simulink model "J8Grav_block"  (R2017b)
settings: Solver=VariableStepAuto  StartTime=0.0  StopTime=10.0  RelTol=1e-3
libraries: sharedtransform x2
settings Model: Creator=mtwal  LastModifiedBy=mtwal

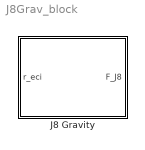
== system J8Grav_block ==
  J8 Gravity : Subsystem  mask(J8 Gravity){w_earth=0, a_earth=0, muE=0, J2_on=on, J3_on=on, J4_on=on, J5_on=on, J6_on=on, J7_on=on, J8_on=on}
      mask prompts: w_earth "Earth rotation rate"; a_earth "Earth semi-major axis"; muE "Earth gravitational parameter"; J2_on "Use J2 harmonic"; J3_on "Use J3 harmonic"; J4_on "Use J4 harmonic"; J5_on "Use J5 harmonic"; J6_on "Use J6 harmonic"; J7_on "Use J7 harmonic"; J8_on "Use J8 harmonic"
      mask help: Calculate force due to J8 gravity from inertial position

== system J8Grav_block/J8 Gravity ==
  r_eci : Inport
  Bus Creator : BusCreator  Inputs=3
  Demux : Demux  Outputs=3
  ECEF2ECI : Subsystem
  ECI2ECEF : Subsystem
  Subsystem : Subsystem
  Subsystem1 : Subsystem
  major axis : Constant  Value=a_earth
  mu : Constant  Value=muE
  F_J8 : Outport
  wires:
  r_eci/1 -> ECI2ECEF/1(v_ECI)
  ECEF2ECI/1(v_ECI) -> F_J8/1  "F_J8_ECI"
  ECI2ECEF/1(v_ECEF) -> Demux/1
  Demux/1 -> Bus Creator/1  "rx"
  Demux/2 -> Bus Creator/2  "ry"
  Demux/3 -> Bus Creator/3  "rz"
  major axis/1 -> Subsystem1/2(a_Earth)  "a_earth"
  mu/1 -> Subsystem1/3(mu_Earth)  "mu_Earth"
  Subsystem/1(J_coeff) -> Subsystem1/4(J_coeff)  "J_coeff"
  Bus Creator/1 -> Subsystem1/1(r_ECEF)  "r_ECEF"
  Subsystem1/1(F_J8Grav_ECEF) -> ECEF2ECI/1(v_ECEF)  "F_J8_ECEF"

== system J8Grav_block/J8 Gravity/ECEF2ECI ==
  v_ECEF : Inport
  Clock : Clock
  Constant : Constant  Value=0
  Gain : Gain  Gain=-w_earth
  Mux : Mux  Inputs=3
  Product : Product  Multiplication=Matrix(*)
  Rotation Angles to Direction Cosine Matrix : sharedtransform/Rotation Angles to Direction Cosine Matrix  rotationOrder=ZYX
      settings: SourceProductBaseCode=AE
  v_ECI : Outport
  wires:
  Clock/1 -> Gain/1
  Gain/1 -> Mux/1
  Product/1 -> v_ECI/1
  Rotation Angles to Direction Cosine Matrix/1 -> Product/1
  v_ECEF/1 -> Product/2
  Mux/1 -> Rotation Angles to Direction Cosine Matrix/1
  Constant/1 -> Mux/2, Mux/3

== system J8Grav_block/J8 Gravity/ECI2ECEF ==
  v_ECI : Inport
  Clock : Clock
  Constant : Constant  Value=0
  Gain : Gain  Gain=w_earth
  Mux : Mux  Inputs=3
  Product : Product  Multiplication=Matrix(*)
  Rotation Angles to Direction Cosine Matrix : sharedtransform/Rotation Angles to Direction Cosine Matrix  rotationOrder=ZYX
      settings: SourceProductBaseCode=AE
  v_ECEF : Outport
  wires:
  Clock/1 -> Gain/1
  Gain/1 -> Mux/1
  Product/1 -> v_ECEF/1
  Rotation Angles to Direction Cosine Matrix/1 -> Product/1
  v_ECI/1 -> Product/2
  Constant/1 -> Mux/2, Mux/3
  Mux/1 -> Rotation Angles to Direction Cosine Matrix/1

== system J8Grav_block/J8 Gravity/Subsystem ==
  Bus Creator : BusCreator  Inputs=7
  J2 : Subsystem
  J3 : Subsystem
  J4 : Subsystem
  J5 : Subsystem
  J6 : Subsystem
  J7 : Subsystem
  J8 : Subsystem
  J_coeff : Outport
  wires:
  J2/1(J2) -> Bus Creator/1  "J2_coeff"
  J3/1(J3) -> Bus Creator/2  "J3_coeff"
  J4/1(J4) -> Bus Creator/3  "J4_coeff"
  J5/1(J5) -> Bus Creator/4  "J5_coeff"
  J6/1(J6) -> Bus Creator/5  "J6_coeff"
  J8/1(J8) -> Bus Creator/7  "J8_coeff"
  J7/1(J7) -> Bus Creator/6  "J7_coeff"
  Bus Creator/1 -> J_coeff/1

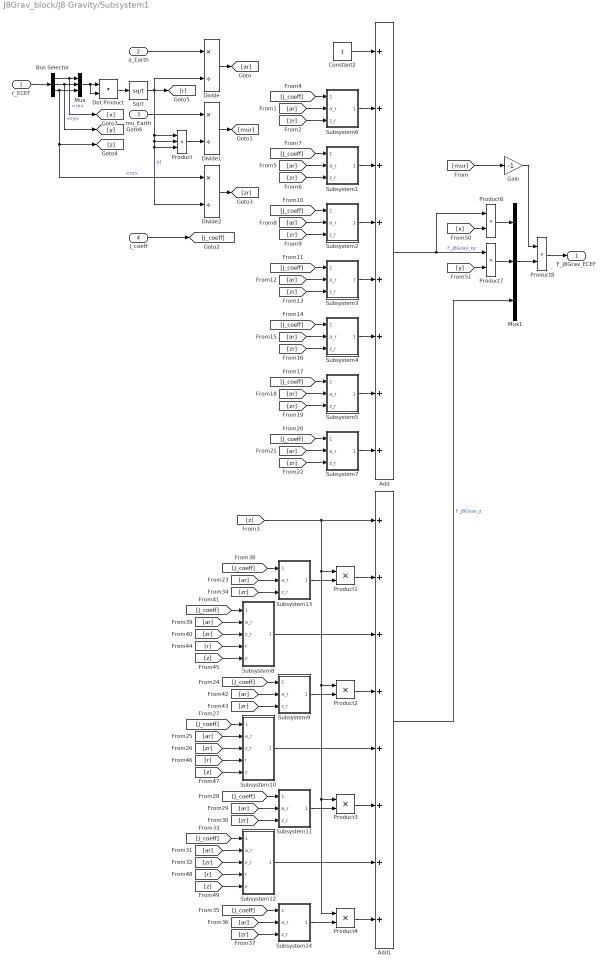
== system J8Grav_block/J8 Gravity/Subsystem1 ==
  r_ECEF : Inport
  a_Earth : Inport  Port=2
  mu_Earth : Inport  Port=3
  J_coeff : Inport  Port=4
  Add : Sum  Inputs=++++++++
  Add1 : Sum  Inputs=++++++++
  Bus Selector : BusSelector  OutputSignals=rx,ry,rz
  Constant2 : Constant
  Divide : Product  Inputs=*/
  Divide1 : Product  Inputs=*/
  Divide2 : Product  Inputs=*/
  Dot Product : DotProduct  InputSameDT=on  OutDataTypeStr=Inherit: Inherit via internal rule
  Gain : Gain  Gain=-1
  Mux : Mux  Inputs=3
  Mux1 : Mux  Inputs=3
  Product : Product  Inputs=3
  Product{1..4,6..8} (7 alike) : Product
  Sqrt : Sqrt  SaturateOnIntegerOverflow=on
  Subsystem1 : Subsystem
  Subsystem10 : Subsystem
  Subsystem11 : Subsystem
  Subsystem12 : Subsystem
  Subsystem13 : Subsystem
  Subsystem14 : Subsystem
  Subsystem2 : Subsystem
  Subsystem3 : Subsystem
  Subsystem4 : Subsystem
  Subsystem5 : Subsystem
  Subsystem6 : Subsystem
  Subsystem7 : Subsystem
  Subsystem8 : Subsystem
  Subsystem9 : Subsystem
  F_J8Grav_ECEF : Outport
  wires:
  r_ECEF/1 -> Bus Selector/1
  Bus Selector/1 -> [x], Mux/1  "<rx>"
  Bus Selector/2 -> [y], Mux/2  "<ry>"
  Bus Selector/3 -> Mux/3, [z], Divide2/1  "<rz>"
  Mux/1 -> Dot Product/2, Dot Product/1
  Dot Product/1 -> Sqrt/1
  Sqrt/1 -> [r], Divide/2, Product/1, Product/2, Product/3, Divide2/2  "|r|"
  a_Earth/1 -> Divide/1
  mu_Earth/1 -> Divide1/1
  Divide/1 -> [ar]
  Divide1/1 -> [mur]
  Product/1 -> Divide1/2
  Divide2/1 -> [zr]
  J_coeff/1 -> [J_coeff]
  [J_coeff] -> Subsystem6/1(J_coeff)
  [ar] -> Subsystem6/2(a_r)
  [zr] -> Subsystem6/3(z_r)
  Subsystem6/1(F_J2_xy) -> Add/2
  Constant2/1 -> Add/1
  Subsystem1/1(F_J3_xy) -> Add/3
  [J_coeff] -> Subsystem1/1(J_coeff)
  [ar] -> Subsystem1/2(a_r)
  [zr] -> Subsystem1/3(z_r)
  Subsystem2/1(F_J4_xy) -> Add/4
  [zr] -> Subsystem2/3(z_r)
  [ar] -> Subsystem2/2(a_r)
  [J_coeff] -> Subsystem2/1(J_coeff)
  [J_coeff] -> Subsystem3/1(J_coeff)
  [ar] -> Subsystem3/2(a_r)
  [zr] -> Subsystem3/3(z_r)
  Subsystem3/1(F_J5_xy) -> Add/5
  [zr] -> Subsystem4/3(z_r)
  [ar] -> Subsystem4/2(a_r)
  [J_coeff] -> Subsystem4/1(J_coeff)
  Subsystem4/1(F_J6_xy) -> Add/6
  [J_coeff] -> Subsystem5/1(J_coeff)
  [zr] -> Subsystem5/3(z_r)
  [ar] -> Subsystem5/2(a_r)
  Subsystem5/1(F_J7_xy) -> Add/7
  [zr] -> Subsystem7/3(z_r)
  [ar] -> Subsystem7/2(a_r)
  [J_coeff] -> Subsystem7/1(J_coeff)
  Subsystem7/1(F_J8_xy) -> Add/8
  Add/1 -> Product6/1, Product7/1  "F_J8Grav_xy"
  [J_coeff] -> Subsystem11/1(J_coeff)
  [zr] -> Subsystem11/3(z_r)
  [J_coeff] -> Subsystem13/1(J_coeff)
  Subsystem8/1(F_J3_z) -> Add1/3
  Subsystem12/1(F_J7_z) -> Add1/7
  Add1/1 -> Mux1/3  "F_J8Grav_z"
  [J_coeff] -> Subsystem8/1(J_coeff)
  [zr] -> Subsystem13/3(z_r)
  [J_coeff] -> Subsystem9/1(J_coeff)
  [ar] -> Subsystem9/2(a_r)
  [zr] -> Subsystem9/3(z_r)
  [ar] -> Subsystem13/2(a_r)
  [zr] -> Subsystem8/3(z_r)
  [J_coeff] -> Subsystem14/1(J_coeff)
  [ar] -> Subsystem11/2(a_r)
  [zr] -> Subsystem14/3(z_r)
  [ar] -> Subsystem14/2(a_r)
  [z] -> Product2/1, Product4/1, Product3/1, Product1/1, Add1/1
  [ar] -> Subsystem8/2(a_r)
  Product1/1 -> Add1/2
  Subsystem13/1(F_J2_z) -> Product1/2
  Product2/1 -> Add1/4
  Subsystem9/1(F_J4_z) -> Product2/2
  Product3/1 -> Add1/6
  Subsystem11/1(F_J6_z) -> Product3/2
  Product4/1 -> Add1/8
  Subsystem14/1(F_J8_xy) -> Product4/2
  [z] -> Subsystem8/5(z)
  [r] -> Subsystem8/4(r)
  [ar] -> Subsystem10/2(a_r)
  [z] -> Subsystem10/5(z)
  [zr] -> Subsystem10/3(z_r)
  [J_coeff] -> Subsystem10/1(J_coeff)
  [r] -> Subsystem10/4(r)
  Subsystem10/1(F_J5_z) -> Add1/5
  [r] -> Subsystem12/4(r)
  [J_coeff] -> Subsystem12/1(J_coeff)
  [zr] -> Subsystem12/3(z_r)
  [ar] -> Subsystem12/2(a_r)
  [z] -> Subsystem12/5(z)
  [y] -> Product7/2
  Product6/1 -> Mux1/1
  [x] -> Product6/2
  Product7/1 -> Mux1/2
  Mux1/1 -> Product8/2
  Product8/1 -> F_J8Grav_ECEF/1
  [mur] -> Gain/1
  Gain/1 -> Product8/1

== system J8Grav_block/J8 Gravity/Subsystem/J2 ==
  Constant : Constant  Value=J2_on
  Constant7 : Constant  Value=0
  J2 value : Constant  Value=1.08263566655E-03
  Switch : Switch  Criteria=u2 > Threshold
  J2 : Outport
  wires:
  Switch/1 -> J2/1
  Constant/1 -> Switch/2
  Constant7/1 -> Switch/3
  J2 value/1 -> Switch/1

== system J8Grav_block/J8 Gravity/Subsystem/J3 ==
  Constant : Constant  Value=J3_on
  Constant7 : Constant  Value=0
  J3 value : Constant  Value=-2.53247369133E-06
  Switch : Switch  Criteria=u2 > Threshold
  J3 : Outport
  wires:
  Switch/1 -> J3/1
  Constant/1 -> Switch/2
  Constant7/1 -> Switch/3
  J3 value/1 -> Switch/1

== system J8Grav_block/J8 Gravity/Subsystem/J4 ==
  Constant : Constant  Value=J4_on
  Constant7 : Constant  Value=0
  J4 value : Constant  Value=-1.61997430578E-06
  Switch : Switch  Criteria=u2 > Threshold
  J4 : Outport
  wires:
  Switch/1 -> J4/1
  Constant/1 -> Switch/2
  Constant7/1 -> Switch/3
  J4 value/1 -> Switch/1

== system J8Grav_block/J8 Gravity/Subsystem/J5 ==
  Constant : Constant  Value=J5_on
  Constant7 : Constant  Value=0
  J5 value : Constant  Value=-2.27905126082E-07
  Switch : Switch  Criteria=u2 > Threshold
  J5 : Outport
  wires:
  Switch/1 -> J5/1
  Constant/1 -> Switch/2
  Constant7/1 -> Switch/3
  J5 value/1 -> Switch/1

== system J8Grav_block/J8 Gravity/Subsystem/J6 ==
  Constant : Constant  Value=J6_on
  Constant7 : Constant  Value=0
  J6 value : Constant  Value=5.40616789940E-07
  Switch : Switch  Criteria=u2 > Threshold
  J6 : Outport
  wires:
  Switch/1 -> J6/1
  Constant/1 -> Switch/2
  Constant7/1 -> Switch/3
  J6 value/1 -> Switch/1

== system J8Grav_block/J8 Gravity/Subsystem/J7 ==
  Constant : Constant  Value=J7_on
  Constant7 : Constant  Value=0
  J7 value : Constant  Value=-3.50522925632E-07
  Switch : Switch  Criteria=u2 > Threshold
  J7 : Outport
  wires:
  Switch/1 -> J7/1
  Constant/1 -> Switch/2
  Constant7/1 -> Switch/3
  J7 value/1 -> Switch/1

== system J8Grav_block/J8 Gravity/Subsystem/J8 ==
  Constant : Constant  Value=J8_on
  Constant7 : Constant  Value=0
  J8 value : Constant  Value=-2.04016767010E-07
  Switch : Switch  Criteria=u2 > Threshold
  J8 : Outport
  wires:
  Switch/1 -> J8/1
  Constant/1 -> Switch/2
  Constant7/1 -> Switch/3
  J8 value/1 -> Switch/1

== system J8Grav_block/J8 Gravity/Subsystem1/Subsystem1 ==
  J_coeff : Inport
  a_r : Inport  Port=2
  z_r : Inport  Port=3
  Bus Selector1 : BusSelector  OutputSignals=J3_coeff
  Constant : Constant  Value=5/2
  Constant1 : Constant  Value=-7
  Constant2 : Constant  Value=3
  Product1 : Product  Inputs=4
  Product2 : Product
  Product3 : Product  Inputs=3
  Product4 : Product  Inputs=3
  Product5 : Product
  Sum : Sum  Inputs=|++
  F_J3_xy : Outport
  wires:
  Sum/1 -> Product1/4
  Product2/1 -> Sum/1
  J_coeff/1 -> Bus Selector1/1
  Bus Selector1/1 -> Product1/2  "<J3_coeff>"
  Constant/1 -> Product1/1
  Constant1/1 -> Product2/1
  Product1/1 -> F_J3_xy/1
  a_r/1 -> Product3/3, Product3/1, Product3/2
  Product3/1 -> Product1/3
  Product4/1 -> Product2/2
  z_r/1 -> Product5/2, Product4/3, Product4/1, Product4/2
  Constant2/1 -> Product5/1
  Product5/1 -> Sum/2

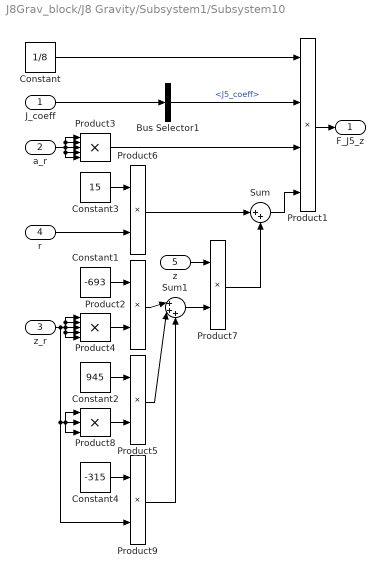
== system J8Grav_block/J8 Gravity/Subsystem1/Subsystem10 ==
  J_coeff : Inport
  a_r : Inport  Port=2
  z_r : Inport  Port=3
  r : Inport  Port=4
  z : Inport  Port=5
  Bus Selector1 : BusSelector  OutputSignals=J5_coeff
  Constant : Constant  Value=1/8
  Constant1 : Constant  Value=-693
  Constant2 : Constant  Value=945
  Constant3 : Constant  Value=15
  Constant4 : Constant  Value=-315
  Product1 : Product  Inputs=4
  Product{2,5..7,9} (5 alike) : Product
  Product3 : Product  Inputs=5
  Product4 : Product  Inputs=5
  Product8 : Product  Inputs=3
  Sum : Sum  Inputs=|++
  Sum1 : Sum  Inputs=|+++
  F_J5_z : Outport
  wires:
  Sum/1 -> Product1/4
  J_coeff/1 -> Bus Selector1/1
  Bus Selector1/1 -> Product1/2  "<J5_coeff>"
  Constant/1 -> Product1/1
  Constant1/1 -> Product2/1
  Product1/1 -> F_J5_z/1
  a_r/1 -> Product3/5, Product3/4, Product3/1, Product3/2, Product3/3
  Product3/1 -> Product1/3
  Product4/1 -> Product2/2
  z_r/1 -> Product9/2, Product8/3, Product8/1, Product8/2, Product4/5, Product4/4, Product4/1, Product4/2, Product4/3
  Constant2/1 -> Product5/1
  Product6/1 -> Sum/1
  r/1 -> Product6/2
  Constant3/1 -> Product6/1
  Product2/1 -> Sum1/1
  Sum1/1 -> Product7/2
  Product5/1 -> Sum1/2
  z/1 -> Product7/1
  Product7/1 -> Sum/2
  Product8/1 -> Product5/2
  Product9/1 -> Sum1/3
  Constant4/1 -> Product9/1

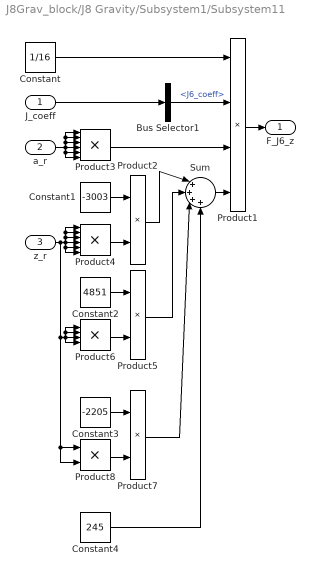
== system J8Grav_block/J8 Gravity/Subsystem1/Subsystem11 ==
  J_coeff : Inport
  a_r : Inport  Port=2
  z_r : Inport  Port=3
  Bus Selector1 : BusSelector  OutputSignals=J6_coeff
  Constant : Constant  Value=1/16
  Constant1 : Constant  Value=-3003
  Constant2 : Constant  Value=4851
  Constant3 : Constant  Value=-2205
  Constant4 : Constant  Value=245
  Product1 : Product  Inputs=4
  Product{2,5,7..8} (4 alike) : Product
  Product3 : Product  Inputs=6
  Product4 : Product  Inputs=6
  Product6 : Product  Inputs=4
  Sum : Sum  Inputs=|++++
  F_J6_z : Outport
  wires:
  Sum/1 -> Product1/4
  Product2/1 -> Sum/1
  J_coeff/1 -> Bus Selector1/1
  Bus Selector1/1 -> Product1/2  "<J6_coeff>"
  Constant/1 -> Product1/1
  Constant1/1 -> Product2/1
  Product1/1 -> F_J6_z/1
  a_r/1 -> Product3/1, Product3/2, Product3/3, Product3/6, Product3/5, Product3/4
  Product3/1 -> Product1/3
  Product4/1 -> Product2/2
  z_r/1 -> Product8/1, Product8/2, Product6/1, Product6/2, Product6/4, Product6/3, Product4/1, Product4/2, Product4/3, Product4/6, Product4/5, Product4/4
  Constant2/1 -> Product5/1
  Product5/1 -> Sum/2
  Product6/1 -> Product5/2
  Constant3/1 -> Product7/1
  Product7/1 -> Sum/3
  Product8/1 -> Product7/2
  Constant4/1 -> Sum/4

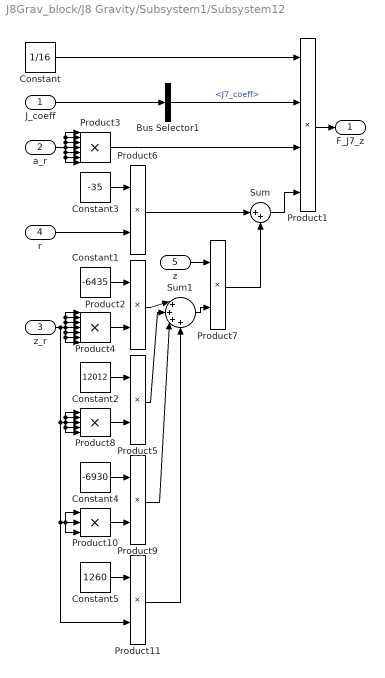
== system J8Grav_block/J8 Gravity/Subsystem1/Subsystem12 ==
  J_coeff : Inport
  a_r : Inport  Port=2
  z_r : Inport  Port=3
  r : Inport  Port=4
  z : Inport  Port=5
  Bus Selector1 : BusSelector  OutputSignals=J7_coeff
  Constant : Constant  Value=1/16
  Constant1 : Constant  Value=-6435
  Constant2 : Constant  Value=12012
  Constant3 : Constant  Value=-35
  Constant4 : Constant  Value=-6930
  Constant5 : Constant  Value=1260
  Product1 : Product  Inputs=4
  Product10 : Product  Inputs=3
  Product{2,5..7,9,11} (6 alike) : Product
  Product3 : Product  Inputs=7
  Product4 : Product  Inputs=7
  Product8 : Product  Inputs=5
  Sum : Sum  Inputs=|++
  Sum1 : Sum  Inputs=|++++
  F_J7_z : Outport
  wires:
  Sum/1 -> Product1/4
  J_coeff/1 -> Bus Selector1/1
  Bus Selector1/1 -> Product1/2  "<J7_coeff>"
  Constant/1 -> Product1/1
  Constant1/1 -> Product2/1
  Product1/1 -> F_J7_z/1
  a_r/1 -> Product3/3, Product3/1, Product3/2, Product3/7, Product3/6, Product3/5, Product3/4
  Product3/1 -> Product1/3
  Product4/1 -> Product2/2
  z_r/1 -> Product11/2, Product10/3, Product10/1, Product10/2, Product8/5, Product8/4, Product8/1, Product8/2, Product8/3, Product4/3, Product4/1, Product4/2, Product4/7, Product4/6, Product4/5, Product4/4
  Constant2/1 -> Product5/1
  Product6/1 -> Sum/1
  r/1 -> Product6/2
  Constant3/1 -> Product6/1
  Product2/1 -> Sum1/1
  Sum1/1 -> Product7/2
  Product5/1 -> Sum1/2
  z/1 -> Product7/1
  Product7/1 -> Sum/2
  Product8/1 -> Product5/2
  Product9/1 -> Sum1/3
  Constant4/1 -> Product9/1
  Product10/1 -> Product9/2
  Constant5/1 -> Product11/1
  Product11/1 -> Sum1/4

== system J8Grav_block/J8 Gravity/Subsystem1/Subsystem13 ==
  J_coeff : Inport
  a_r : Inport  Port=2
  z_r : Inport  Port=3
  Bus Selector1 : BusSelector  OutputSignals=J2_coeff
  Constant : Constant  Value=3/2
  Constant1 : Constant  Value=-5
  Constant2 : Constant  Value=3
  Product1 : Product  Inputs=4
  Product2 : Product
  Product3 : Product
  Product4 : Product
  Sum : Sum  Inputs=|++
  F_J2_z : Outport
  wires:
  Sum/1 -> Product1/4
  Product2/1 -> Sum/1
  J_coeff/1 -> Bus Selector1/1
  Bus Selector1/1 -> Product1/2  "<J2_coeff>"
  Constant/1 -> Product1/1
  Constant1/1 -> Product2/1
  Product1/1 -> F_J2_z/1
  a_r/1 -> Product3/1, Product3/2
  Product3/1 -> Product1/3
  Product4/1 -> Product2/2
  z_r/1 -> Product4/1, Product4/2
  Constant2/1 -> Sum/2

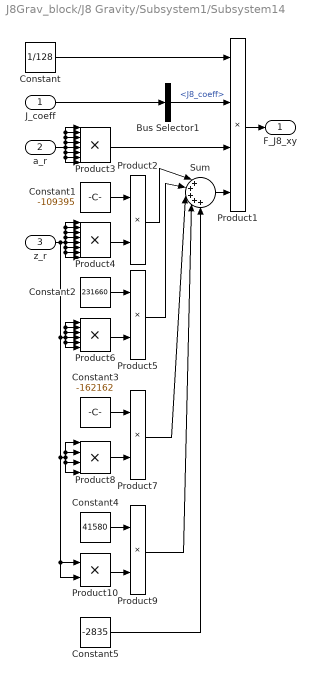
== system J8Grav_block/J8 Gravity/Subsystem1/Subsystem14 ==
  J_coeff : Inport
  a_r : Inport  Port=2
  z_r : Inport  Port=3
  Bus Selector1 : BusSelector  OutputSignals=J8_coeff
  Constant : Constant  Value=1/128
  Constant1 : Constant  Value=-109395
  Constant2 : Constant  Value=231660
  Constant3 : Constant  Value=-162162
  Constant4 : Constant  Value=41580
  Constant5 : Constant  Value=-2835
  Product1 : Product  Inputs=4
  Product{2,5,7,9..10} (5 alike) : Product
  Product3 : Product  Inputs=8
  Product4 : Product  Inputs=8
  Product6 : Product  Inputs=6
  Product8 : Product  Inputs=4
  Sum : Sum  Inputs=|+++++
  F_J8_xy : Outport
  wires:
  Sum/1 -> Product1/4
  Product2/1 -> Sum/1
  J_coeff/1 -> Bus Selector1/1
  Bus Selector1/1 -> Product1/2  "<J8_coeff>"
  Constant/1 -> Product1/1
  Constant1/1 -> Product2/1
  Product1/1 -> F_J8_xy/1
  a_r/1 -> Product3/1, Product3/2, Product3/3, Product3/4, Product3/8, Product3/7, Product3/6, Product3/5
  Product3/1 -> Product1/3
  Product4/1 -> Product2/2
  z_r/1 -> Product10/2, Product10/1, Product8/1, Product8/2, Product8/4, Product8/3, Product6/1, Product6/2, Product6/3, Product6/6, Product6/5, Product6/4, Product4/1, Product4/2, Product4/3, Product4/4, Product4/8, Product4/7, Product4/6, Product4/5
  Constant2/1 -> Product5/1
  Product5/1 -> Sum/2
  Product6/1 -> Product5/2
  Constant3/1 -> Product7/1
  Product7/1 -> Sum/3
  Product8/1 -> Product7/2
  Constant4/1 -> Product9/1
  Product9/1 -> Sum/4
  Product10/1 -> Product9/2
  Constant5/1 -> Sum/5

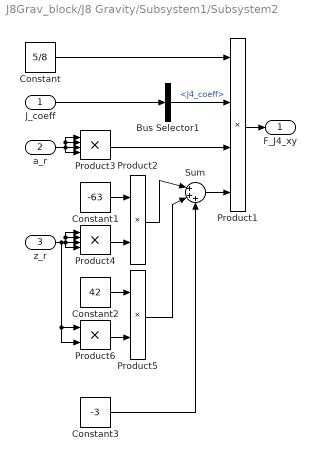
== system J8Grav_block/J8 Gravity/Subsystem1/Subsystem2 ==
  J_coeff : Inport
  a_r : Inport  Port=2
  z_r : Inport  Port=3
  Bus Selector1 : BusSelector  OutputSignals=J4_coeff
  Constant : Constant  Value=5/8
  Constant1 : Constant  Value=-63
  Constant2 : Constant  Value=42
  Constant3 : Constant  Value=-3
  Product1 : Product  Inputs=4
  Product2 : Product
  Product3 : Product  Inputs=4
  Product4 : Product  Inputs=4
  Product5 : Product
  Product6 : Product
  Sum : Sum  Inputs=|+++
  F_J4_xy : Outport
  wires:
  Sum/1 -> Product1/4
  Product2/1 -> Sum/1
  J_coeff/1 -> Bus Selector1/1
  Bus Selector1/1 -> Product1/2  "<J4_coeff>"
  Constant/1 -> Product1/1
  Constant1/1 -> Product2/1
  Product1/1 -> F_J4_xy/1
  a_r/1 -> Product3/4, Product3/1, Product3/2, Product3/3
  Product3/1 -> Product1/3
  Product4/1 -> Product2/2
  z_r/1 -> Product6/2, Product6/1, Product4/1, Product4/2, Product4/4, Product4/3
  Constant2/1 -> Product5/1
  Product5/1 -> Sum/2
  Product6/1 -> Product5/2
  Constant3/1 -> Sum/3

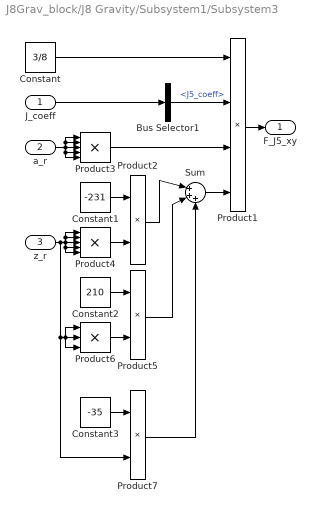
== system J8Grav_block/J8 Gravity/Subsystem1/Subsystem3 ==
  J_coeff : Inport
  a_r : Inport  Port=2
  z_r : Inport  Port=3
  Bus Selector1 : BusSelector  OutputSignals=J5_coeff
  Constant : Constant  Value=3/8
  Constant1 : Constant  Value=-231
  Constant2 : Constant  Value=210
  Constant3 : Constant  Value=-35
  Product1 : Product  Inputs=4
  Product2 : Product
  Product3 : Product  Inputs=5
  Product4 : Product  Inputs=5
  Product5 : Product
  Product6 : Product  Inputs=3
  Product7 : Product
  Sum : Sum  Inputs=|+++
  F_J5_xy : Outport
  wires:
  Sum/1 -> Product1/4
  Product2/1 -> Sum/1
  J_coeff/1 -> Bus Selector1/1
  Bus Selector1/1 -> Product1/2  "<J5_coeff>"
  Constant/1 -> Product1/1
  Constant1/1 -> Product2/1
  Product1/1 -> F_J5_xy/1
  a_r/1 -> Product3/5, Product3/4, Product3/1, Product3/2, Product3/3
  Product3/1 -> Product1/3
  Product4/1 -> Product2/2
  z_r/1 -> Product7/2, Product6/3, Product6/1, Product6/2, Product4/1, Product4/2, Product4/5, Product4/4, Product4/3
  Constant2/1 -> Product5/1
  Product5/1 -> Sum/2
  Product6/1 -> Product5/2
  Constant3/1 -> Product7/1
  Product7/1 -> Sum/3

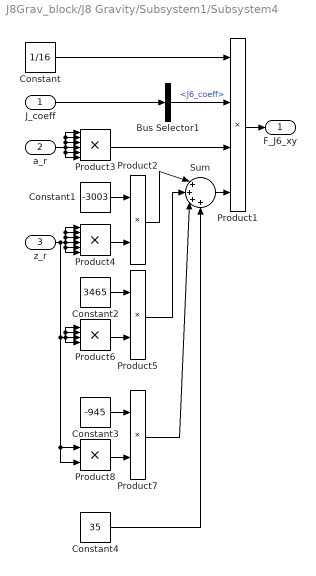
== system J8Grav_block/J8 Gravity/Subsystem1/Subsystem4 ==
  J_coeff : Inport
  a_r : Inport  Port=2
  z_r : Inport  Port=3
  Bus Selector1 : BusSelector  OutputSignals=J6_coeff
  Constant : Constant  Value=1/16
  Constant1 : Constant  Value=-3003
  Constant2 : Constant  Value=3465
  Constant3 : Constant  Value=-945
  Constant4 : Constant  Value=35
  Product1 : Product  Inputs=4
  Product{2,5,7..8} (4 alike) : Product
  Product3 : Product  Inputs=6
  Product4 : Product  Inputs=6
  Product6 : Product  Inputs=4
  Sum : Sum  Inputs=|++++
  F_J6_xy : Outport
  wires:
  Sum/1 -> Product1/4
  Product2/1 -> Sum/1
  J_coeff/1 -> Bus Selector1/1
  Bus Selector1/1 -> Product1/2  "<J6_coeff>"
  Constant/1 -> Product1/1
  Constant1/1 -> Product2/1
  Product1/1 -> F_J6_xy/1
  a_r/1 -> Product3/1, Product3/2, Product3/3, Product3/6, Product3/5, Product3/4
  Product3/1 -> Product1/3
  Product4/1 -> Product2/2
  z_r/1 -> Product8/1, Product8/2, Product6/1, Product6/2, Product6/4, Product6/3, Product4/1, Product4/2, Product4/3, Product4/6, Product4/5, Product4/4
  Constant2/1 -> Product5/1
  Product5/1 -> Sum/2
  Product6/1 -> Product5/2
  Constant3/1 -> Product7/1
  Product7/1 -> Sum/3
  Product8/1 -> Product7/2
  Constant4/1 -> Sum/4

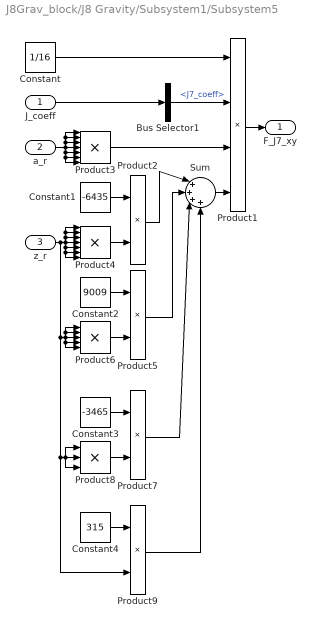
== system J8Grav_block/J8 Gravity/Subsystem1/Subsystem5 ==
  J_coeff : Inport
  a_r : Inport  Port=2
  z_r : Inport  Port=3
  Bus Selector1 : BusSelector  OutputSignals=J7_coeff
  Constant : Constant  Value=1/16
  Constant1 : Constant  Value=-6435
  Constant2 : Constant  Value=9009
  Constant3 : Constant  Value=-3465
  Constant4 : Constant  Value=315
  Product1 : Product  Inputs=4
  Product{2,5,7,9} (4 alike) : Product
  Product3 : Product  Inputs=7
  Product4 : Product  Inputs=7
  Product6 : Product  Inputs=5
  Product8 : Product  Inputs=3
  Sum : Sum  Inputs=|++++
  F_J7_xy : Outport
  wires:
  Sum/1 -> Product1/4
  Product2/1 -> Sum/1
  J_coeff/1 -> Bus Selector1/1
  Bus Selector1/1 -> Product1/2  "<J7_coeff>"
  Constant/1 -> Product1/1
  Constant1/1 -> Product2/1
  Product1/1 -> F_J7_xy/1
  a_r/1 -> Product3/1, Product3/2, Product3/3, Product3/7, Product3/6, Product3/5, Product3/4
  Product3/1 -> Product1/3
  Product4/1 -> Product2/2
  z_r/1 -> Product9/2, Product8/3, Product8/1, Product8/2, Product6/1, Product6/2, Product6/5, Product6/4, Product6/3, Product4/1, Product4/2, Product4/3, Product4/7, Product4/6, Product4/5, Product4/4
  Constant2/1 -> Product5/1
  Product5/1 -> Sum/2
  Product6/1 -> Product5/2
  Constant3/1 -> Product7/1
  Product7/1 -> Sum/3
  Product8/1 -> Product7/2
  Constant4/1 -> Product9/1
  Product9/1 -> Sum/4

== system J8Grav_block/J8 Gravity/Subsystem1/Subsystem6 ==
  J_coeff : Inport
  a_r : Inport  Port=2
  z_r : Inport  Port=3
  Bus Selector1 : BusSelector  OutputSignals=J2_coeff
  Constant : Constant  Value=3/2
  Constant1 : Constant  Value=-5
  Constant2 : Constant
  Product1 : Product  Inputs=4
  Product2 : Product
  Product3 : Product
  Product4 : Product
  Sum : Sum  Inputs=|++
  F_J2_xy : Outport
  wires:
  Sum/1 -> Product1/4
  Product2/1 -> Sum/1
  J_coeff/1 -> Bus Selector1/1
  Bus Selector1/1 -> Product1/2  "<J2_coeff>"
  Constant/1 -> Product1/1
  Constant1/1 -> Product2/1
  Product1/1 -> F_J2_xy/1
  a_r/1 -> Product3/1, Product3/2
  Product3/1 -> Product1/3
  Product4/1 -> Product2/2
  z_r/1 -> Product4/1, Product4/2
  Constant2/1 -> Sum/2

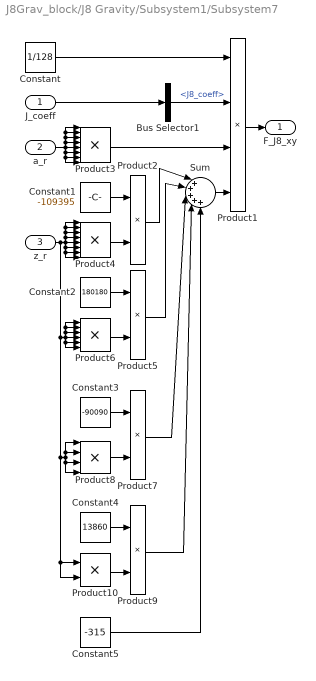
== system J8Grav_block/J8 Gravity/Subsystem1/Subsystem7 ==
  J_coeff : Inport
  a_r : Inport  Port=2
  z_r : Inport  Port=3
  Bus Selector1 : BusSelector  OutputSignals=J8_coeff
  Constant : Constant  Value=1/128
  Constant1 : Constant  Value=-109395
  Constant2 : Constant  Value=180180
  Constant3 : Constant  Value=-90090
  Constant4 : Constant  Value=13860
  Constant5 : Constant  Value=-315
  Product1 : Product  Inputs=4
  Product{2,5,7,9..10} (5 alike) : Product
  Product3 : Product  Inputs=8
  Product4 : Product  Inputs=8
  Product6 : Product  Inputs=6
  Product8 : Product  Inputs=4
  Sum : Sum  Inputs=|+++++
  F_J8_xy : Outport
  wires:
  Sum/1 -> Product1/4
  Product2/1 -> Sum/1
  J_coeff/1 -> Bus Selector1/1
  Bus Selector1/1 -> Product1/2  "<J8_coeff>"
  Constant/1 -> Product1/1
  Constant1/1 -> Product2/1
  Product1/1 -> F_J8_xy/1
  a_r/1 -> Product3/1, Product3/2, Product3/3, Product3/4, Product3/8, Product3/7, Product3/6, Product3/5
  Product3/1 -> Product1/3
  Product4/1 -> Product2/2
  z_r/1 -> Product10/2, Product10/1, Product8/1, Product8/2, Product8/4, Product8/3, Product6/1, Product6/2, Product6/3, Product6/6, Product6/5, Product6/4, Product4/1, Product4/2, Product4/3, Product4/4, Product4/8, Product4/7, Product4/6, Product4/5
  Constant2/1 -> Product5/1
  Product5/1 -> Sum/2
  Product6/1 -> Product5/2
  Constant3/1 -> Product7/1
  Product7/1 -> Sum/3
  Product8/1 -> Product7/2
  Constant4/1 -> Product9/1
  Product9/1 -> Sum/4
  Product10/1 -> Product9/2
  Constant5/1 -> Sum/5

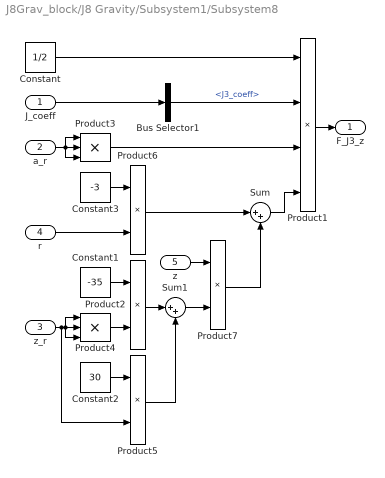
== system J8Grav_block/J8 Gravity/Subsystem1/Subsystem8 ==
  J_coeff : Inport
  a_r : Inport  Port=2
  z_r : Inport  Port=3
  r : Inport  Port=4
  z : Inport  Port=5
  Bus Selector1 : BusSelector  OutputSignals=J3_coeff
  Constant : Constant  Value=1/2
  Constant1 : Constant  Value=-35
  Constant2 : Constant  Value=30
  Constant3 : Constant  Value=-3
  Product1 : Product  Inputs=4
  Product{2,5..7} (4 alike) : Product
  Product3 : Product  Inputs=3
  Product4 : Product  Inputs=3
  Sum : Sum  Inputs=|++
  Sum1 : Sum  Inputs=|++
  F_J3_z : Outport
  wires:
  Sum/1 -> Product1/4
  J_coeff/1 -> Bus Selector1/1
  Bus Selector1/1 -> Product1/2  "<J3_coeff>"
  Constant/1 -> Product1/1
  Constant1/1 -> Product2/1
  Product1/1 -> F_J3_z/1
  a_r/1 -> Product3/3, Product3/1, Product3/2
  Product3/1 -> Product1/3
  Product4/1 -> Product2/2
  z_r/1 -> Product5/2, Product4/3, Product4/1, Product4/2
  Constant2/1 -> Product5/1
  Product6/1 -> Sum/1
  r/1 -> Product6/2
  Constant3/1 -> Product6/1
  Product2/1 -> Sum1/1
  Sum1/1 -> Product7/2
  Product5/1 -> Sum1/2
  z/1 -> Product7/1
  Product7/1 -> Sum/2

== system J8Grav_block/J8 Gravity/Subsystem1/Subsystem9 ==
  J_coeff : Inport
  a_r : Inport  Port=2
  z_r : Inport  Port=3
  Bus Selector1 : BusSelector  OutputSignals=J4_coeff
  Constant : Constant  Value=5/8
  Constant1 : Constant  Value=-63
  Constant2 : Constant  Value=70
  Constant3 : Constant  Value=-15
  Product1 : Product  Inputs=4
  Product2 : Product
  Product3 : Product  Inputs=4
  Product4 : Product  Inputs=4
  Product5 : Product
  Product6 : Product
  Sum : Sum  Inputs=|+++
  F_J4_z : Outport
  wires:
  Sum/1 -> Product1/4
  Product2/1 -> Sum/1
  J_coeff/1 -> Bus Selector1/1
  Bus Selector1/1 -> Product1/2  "<J4_coeff>"
  Constant/1 -> Product1/1
  Constant1/1 -> Product2/1
  Product1/1 -> F_J4_z/1
  a_r/1 -> Product3/4, Product3/1, Product3/2, Product3/3
  Product3/1 -> Product1/3
  Product4/1 -> Product2/2
  z_r/1 -> Product6/2, Product6/1, Product4/1, Product4/2, Product4/4, Product4/3
  Constant2/1 -> Product5/1
  Product5/1 -> Sum/2
  Product6/1 -> Product5/2
  Constant3/1 -> Sum/3
